simulink model "mod_5_counter"  (R2020a)
settings: Solver=VariableStepAuto  StartTime=0.0  StopTime=10.0  RelTol=1e-3
settings Model: Creator=USER  LastModifiedBy=USER

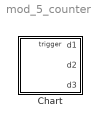
== system mod_5_counter ==
  Chart : Stateflow chart  TreatAsAtomicUnit=on

== stateflow chart mod_5_counter/Chart ==
  state State_0
    state digit2
      en:d2=0;
    state digit1
      en:d1=0;
    state digit3
      en:d3=0;
    State_0.digit1 -> State_0.digit2 : clk
    State_0.digit2 -> State_0.digit3 : clk
    (default) -> State_0.digit1
    State_0.digit3 -> State_0.digit1 : clk/{clk1}
  state State_1
    state digit2
      en:d2=0;
    state digit1
      en:d1=0;
    state digit3
      en:d3=1;
    State_1.digit1 -> State_1.digit2 : clk1
    State_1.digit2 -> State_1.digit3 : clk1
    (default) -> State_1.digit1
    State_1.digit3 -> State_1.digit1 : clk1
  state State_2
    state digit2
      en:d2=1;
    state digit1
      en:d1=0;
    state digit3
      en:d3=0;
    State_2.digit1 -> State_2.digit2 : clk2
    State_2.digit2 -> State_2.digit3 : clk2
    (default) -> State_2.digit1
    State_2.digit3 -> State_2.digit1 : clk2/{clk3}
  state digit2
    en:d2=1;
  state digit3
    en:d3=1;
  state digit1
    en:d1=0;
  digit2 -> digit3 : clk3
  digit1 -> digit2 : clk3
  (default) -> digit1
  digit3 -> digit1 : clk3/{clk4}
  data: d1 output; d2 output; d3 output
  events: clk input RISING_EDGE_EVENT; clk1 local RISING_EDGE_EVENT; clk2 local FUNCTION_CALL_EVENT; clk3 local FUNCTION_CALL_EVENT
